simulink model "two_point_four"  (R2014b)
settings: Solver=ode45  StartTime=0.0  StopTime=20  MaxStep=0.001  RelTol=1e-3
values from neighbouring files (symbols this model uses):
  Td = []    [Sint_Bode (4).m]    (also in Sint_Bode.m)
  Tn = []    [Sint_Bode (4).m]    (also in Sint_Bode.m)
settings Model: Creator=maksimka  LastModifiedBy=maksimka

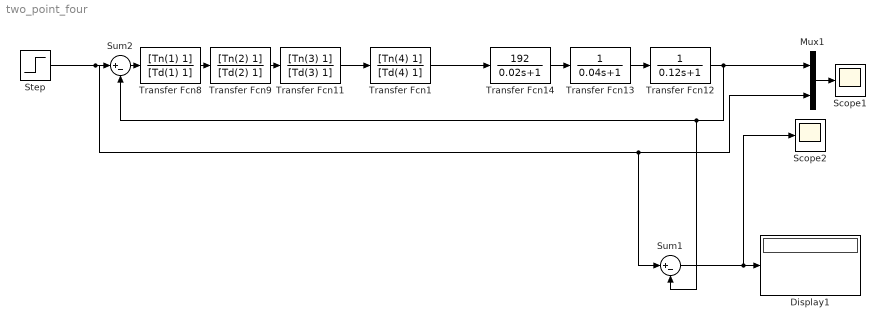
== system two_point_four ==
  Display1 : Display
  Mux1 : Mux  Inputs=2
  Scope1 : Scope
  Scope2 : Scope
      settings: SaveName=ScopeData2  MaxDataPoints=50000
  Step : Step  SampleTime=0
  Sum1 : Sum  Inputs=|+-
  Sum2 : Sum  Inputs=|+-
  Transfer Fcn1 : TransferFcn  Numerator=[Tn(4) 1]  Denominator=[Td(4) 1]
  Transfer Fcn11 : TransferFcn  Numerator=[Tn(3) 1]  Denominator=[Td(3) 1]
  Transfer Fcn12 : TransferFcn  Denominator=[0.12 1]
  Transfer Fcn13 : TransferFcn  Denominator=[0.04 1]
  Transfer Fcn14 : TransferFcn  Numerator=[192]  Denominator=[0.02 1]
  Transfer Fcn8 : TransferFcn  Numerator=[Tn(1) 1]  Denominator=[Td(1) 1]
  Transfer Fcn9 : TransferFcn  Numerator=[Tn(2) 1]  Denominator=[Td(2) 1]
  wires:
  Transfer Fcn8/1 -> Transfer Fcn9/1
  Transfer Fcn9/1 -> Transfer Fcn11/1
  Sum2/1 -> Transfer Fcn8/1
  Transfer Fcn13/1 -> Transfer Fcn12/1
  Transfer Fcn14/1 -> Transfer Fcn13/1
  Transfer Fcn12/1 -> Mux1/1, Sum2/2, Sum1/2
  Mux1/1 -> Scope1/1
  Step/1 -> Sum1/1, Mux1/2, Sum2/1
  Sum1/1 -> Scope2/1, Display1/1
  Transfer Fcn11/1 -> Transfer Fcn1/1
  Transfer Fcn1/1 -> Transfer Fcn14/1
